simulink library "HEMERO"  (Simulink 3.00)
values from neighbouring files (symbols this model uses):
  K1 = 0.5    [ejh64.m]    (also in ejh65.m)
  K2 = 0.8    [ejh64.m]    (also in ejh65.m)
  x_camino = 0:0.01:10    [ejh64.m]    (also in ejh65.m)
  y_camino = x_camino.^2    [ejh64.m]    (also in ejh65.m)
undefined symbols (not defined in the file or in its folder): magnitude, nonlinear
libraries: simulink_extras x12, HEMERO x9, simulink3 x6, dspstat x4
(part 6 of 9)

== system HEMERO/Robots móviles/Control de robots móviles/Métodos basados en Teoría de Control/Seguimiento de trayectorias/Ejemplos/Ejemplo H.6.6/Seguimiento de trayectorias (Control lineal) ==
  note: w
  note: v
  v_r : Inport  Port=1  PortWidth=-1  SampleTime=-1  DataType=auto
      settings: SignalType=auto
  w_r : Inport  Port=2  PortWidth=-1  SampleTime=-1  DataType=auto
      settings: SignalType=auto
  Cambio de variable : Subsystem
  Configuración síncrona referencia : Subsystem
  Configuración síncrona robot real : Subsystem
  Control lineal : Subsystem
  Product : Product  Inputs=2  SaturateOnIntegerOverflow=on
  Sum : Sum  Inputs=-+  SaturateOnIntegerOverflow=on
  Sum1 : Sum  Inputs=+-  SaturateOnIntegerOverflow=on
  Trigonometric Function : Trigonometry  Operator=cos  OutputSignalType=auto
  v : Outport  Orientation=left  Port=1
  w : Outport  Orientation=left  Port=2
  x_ref : Outport  Port=3
  x : Outport  Port=4
  y_ref : Outport  Port=5
  y : Outport  Port=6
  phi_ref : Outport  Port=7
  phi : Outport  Port=8
  wires:
  Configuración síncrona robot real/3(phi) -> phi/1, Cambio de variable/6(phi)
  Configuración síncrona referencia/3(phi_r) -> phi_ref/1, Cambio de variable/5(phi_r)
  Configuración síncrona robot real/2(y) -> y/1, Cambio de variable/4(y)
  Configuración síncrona referencia/2(y_r) -> y_ref/1, Cambio de variable/3(y_r)
  Configuración síncrona robot real/1(x) -> x/1, Cambio de variable/2(x)
  Configuración síncrona referencia/1(x_r) -> x_ref/1, Cambio de variable/1(x_r)
  Cambio de variable/3(e3) -> Control lineal/3(e3), Trigonometric Function/1
  Cambio de variable/2(e2) -> Control lineal/2(e2)
  Cambio de variable/1(e1) -> Control lineal/1(e1)
  Control lineal/1(u1) -> Sum/1
  Control lineal/2(u2) -> Sum1/2
  Sum/1 -> v/1, Configuración síncrona robot real/1(v)
  Sum1/1 -> w/1, Configuración síncrona robot real/2(w)
  w_r/1 -> Sum1/1, Configuración síncrona referencia/2(w_r)
  Product/1 -> Sum/2
  Trigonometric Function/1 -> Product/1
  v_r/1 -> Control lineal/4(v_r), Product/2, Configuración síncrona referencia/1(v_r)

== system HEMERO/Robots móviles/Control de robots móviles/Métodos basados en Teoría de Control/Seguimiento de trayectorias/Ejemplos/Ejemplo H.6.7/Seguimiento de trayectorias (Control lineal con escalado de velocidad) ==
  note: v
  note: w
  v_r : Inport  Port=1  PortWidth=-1  SampleTime=-1  DataType=auto
      settings: SignalType=auto
  w_r : Inport  Port=2  PortWidth=-1  SampleTime=-1  DataType=auto
      settings: SignalType=auto
  Cambio de variable : Subsystem
  Configuración síncrona referencia : Subsystem
  Configuración síncrona robot real : Subsystem
  Control lineal con escalado de velocidad : Subsystem
  Product : Product  Inputs=2  SaturateOnIntegerOverflow=on
  Sum : Sum  Inputs=-+  SaturateOnIntegerOverflow=on
  Sum1 : Sum  Inputs=+-  SaturateOnIntegerOverflow=on
  Trigonometric Function : Trigonometry  Operator=cos  OutputSignalType=auto
  v : Outport  Orientation=left  Port=1
  w : Outport  Orientation=left  Port=2
  x_ref : Outport  Port=3
  x : Outport  Port=4
  y_ref : Outport  Port=5
  y : Outport  Port=6
  phi_ref : Outport  Port=7
  phi : Outport  Port=8
  wires:
  v_r/1 -> Configuración síncrona referencia/1(v_r), Product/2, Control lineal con escalado de velocidad/4(v_r)
  Trigonometric Function/1 -> Product/1
  Product/1 -> Sum/2
  w_r/1 -> Configuración síncrona referencia/2(w_r), Sum1/1, Control lineal con escalado de velocidad/5(w_r)
  Sum1/1 -> Configuración síncrona robot real/2(w), w/1
  Sum/1 -> Configuración síncrona robot real/1(v), v/1
  Control lineal con escalado de velocidad/2(u2) -> Sum1/2
  Control lineal con escalado de velocidad/1(u1) -> Sum/1
  Cambio de variable/1(e1) -> Control lineal con escalado de velocidad/1(e1)
  Cambio de variable/2(e2) -> Control lineal con escalado de velocidad/2(e2)
  Cambio de variable/3(e3) -> Trigonometric Function/1, Control lineal con escalado de velocidad/3(e3)
  Configuración síncrona robot real/3(phi) -> Cambio de variable/6(phi), phi/1
  Configuración síncrona referencia/3(phi_r) -> Cambio de variable/5(phi_r), phi_ref/1
  Configuración síncrona robot real/2(y) -> Cambio de variable/4(y), y/1
  Configuración síncrona referencia/2(y_r) -> Cambio de variable/3(y_r), y_ref/1
  Configuración síncrona robot real/1(x) -> Cambio de variable/2(x), x/1
  Configuración síncrona referencia/1(x_r) -> Cambio de variable/1(x_r), x_ref/1

== system HEMERO/Robots móviles/Control de robots móviles/Métodos basados en Teoría de Control/Seguimiento de trayectorias/Ejemplos/Ejemplo H.6.8/Seguimiento de trayectorias (Control no lineal) ==
  note: v
  note: w
  v_r : Inport  Port=1  PortWidth=-1  SampleTime=-1  DataType=auto
      settings: SignalType=auto
  w_r : Inport  Port=2  PortWidth=-1  SampleTime=-1  DataType=auto
      settings: SignalType=auto
  " " : Trigonometry  Operator=cos  OutputSignalType=auto
  Cambio de variable : Subsystem
  Configuración síncrona referencia : Subsystem
  Configuración síncrona robot real : Subsystem
  Control no lineal : Subsystem
  Cálculo de K1 y K3 : Subsystem
  Product : Product  Inputs=2  SaturateOnIntegerOverflow=on
  Sum : Sum  Inputs=-+  SaturateOnIntegerOverflow=on
  Sum1 : Sum  Inputs=+-  SaturateOnIntegerOverflow=on
  v : Outport  Orientation=left  Port=1
  w : Outport  Orientation=left  Port=2
  x_ref : Outport  Port=3
  x : Outport  Port=4
  y_ref : Outport  Port=5
  y : Outport  Port=6
  phi_ref : Outport  Port=7
  phi : Outport  Port=8
  wires:
  v_r/1 -> Configuración síncrona referencia/1(v_r), Product/2, Control no lineal/4(v_r), Cálculo de K1 y K3/2(v_r)
  " "/1 -> Product/1
  Product/1 -> Sum/2
  w_r/1 -> Configuración síncrona referencia/2(w_r), Sum1/1, Cálculo de K1 y K3/1(w_r)
  Sum1/1 -> Configuración síncrona robot real/2(w), w/1
  Sum/1 -> Configuración síncrona robot real/1(v), v/1
  Control no lineal/2(u2) -> Sum1/2
  Control no lineal/1(u1) -> Sum/1
  Cambio de variable/1(e1) -> Control no lineal/1(e1)
  Cambio de variable/2(e2) -> Control no lineal/2(e2)
  Cambio de variable/3(e3) -> " "/1, Control no lineal/3(e3)
  Cálculo de K1 y K3/1(K1) -> Control no lineal/5(K1), Control no lineal/6(K3)
  Configuración síncrona robot real/3(phi) -> Cambio de variable/6(phi), phi/1
  Configuración síncrona referencia/1(x_r) -> Cambio de variable/1(x_r), x_ref/1
  Configuración síncrona robot real/1(x) -> Cambio de variable/2(x), x/1
  Configuración síncrona referencia/2(y_r) -> Cambio de variable/3(y_r), y_ref/1
  Configuración síncrona robot real/2(y) -> Cambio de variable/4(y), y/1
  Configuración síncrona referencia/3(phi_r) -> Cambio de variable/5(phi_r), phi_ref/1

== system HEMERO/Robots móviles/Control de robots móviles/Métodos basados en Teoría de Control/Seguimiento de trayectorias/Seguimiento de trayectorias (Control lineal con escalado de velocidad)/Cambio de variable/Cálculo de e1 ==
  x_r : Inport  Port=1  PortWidth=-1  SampleTime=-1  DataType=auto
      settings: SignalType=auto
  x : Inport  Port=2  PortWidth=-1  SampleTime=-1  DataType=auto
      settings: SignalType=auto
  y_r : Inport  Port=3  PortWidth=-1  SampleTime=-1  DataType=auto
      settings: SignalType=auto
  y : Inport  Port=4  PortWidth=-1  SampleTime=-1  DataType=auto
      settings: SignalType=auto
  phi : Inport  Port=5  PortWidth=-1  SampleTime=-1  DataType=auto
      settings: SignalType=auto
  Product : Product  Inputs=2  SaturateOnIntegerOverflow=on
  Product1 : Product  Inputs=2  SaturateOnIntegerOverflow=on
  Sum : Sum  Inputs=-+  SaturateOnIntegerOverflow=on
  Sum1 : Sum  Inputs=+-  SaturateOnIntegerOverflow=on
  Sum2 : Sum  Inputs=++  SaturateOnIntegerOverflow=on
  Trigonometric Function : Trigonometry  Operator=sin  OutputSignalType=auto
  Trigonometric Function1 : Trigonometry  Operator=cos  OutputSignalType=auto
  e1 : Outport  Port=1
  wires:
  Sum2/1 -> e1/1
  Product1/1 -> Sum2/2
  Product/1 -> Sum2/1
  Trigonometric Function1/1 -> Product1/2
  Sum1/1 -> Product1/1
  Trigonometric Function/1 -> Product/2
  Sum/1 -> Product/1
  phi/1 -> Trigonometric Function1/1, Trigonometric Function/1
  y/1 -> Sum1/2
  y_r/1 -> Sum1/1
  x/1 -> Sum/2
  x_r/1 -> Sum/1

== system HEMERO/Robots móviles/Control de robots móviles/Métodos basados en Teoría de Control/Seguimiento de trayectorias/Seguimiento de trayectorias (Control lineal con escalado de velocidad)/Cambio de variable/Cálculo de e2 ==
  x_r : Inport  Port=1  PortWidth=-1  SampleTime=-1  DataType=auto
      settings: SignalType=auto
  x : Inport  Port=2  PortWidth=-1  SampleTime=-1  DataType=auto
      settings: SignalType=auto
  y_r : Inport  Port=3  PortWidth=-1  SampleTime=-1  DataType=auto
      settings: SignalType=auto
  y : Inport  Port=4  PortWidth=-1  SampleTime=-1  DataType=auto
      settings: SignalType=auto
  phi : Inport  Port=5  PortWidth=-1  SampleTime=-1  DataType=auto
      settings: SignalType=auto
  Product : Product  Inputs=2  SaturateOnIntegerOverflow=on
  Product1 : Product  Inputs=2  SaturateOnIntegerOverflow=on
  Sum : Sum  Inputs=-+  SaturateOnIntegerOverflow=on
  Sum1 : Sum  Inputs=-+  SaturateOnIntegerOverflow=on
  Sum2 : Sum  Inputs=++  SaturateOnIntegerOverflow=on
  Trigonometric Function2 : Trigonometry  Operator=sin  OutputSignalType=auto
  Trigonometric Function3 : Trigonometry  Operator=cos  OutputSignalType=auto
  e2 : Outport  Port=1
  wires:
  Sum2/1 -> e2/1
  Product1/1 -> Sum2/2
  Product/1 -> Sum2/1
  Trigonometric Function2/1 -> Product1/2
  Sum1/1 -> Product1/1
  Trigonometric Function3/1 -> Product/2
  Sum/1 -> Product/1
  phi/1 -> Trigonometric Function2/1, Trigonometric Function3/1
  y/1 -> Sum1/2
  y_r/1 -> Sum1/1
  x/1 -> Sum/2
  x_r/1 -> Sum/1

== system HEMERO/Robots móviles/Control de robots móviles/Métodos basados en Teoría de Control/Seguimiento de trayectorias/Seguimiento de trayectorias (Control lineal con escalado de velocidad)/Cambio de variable/Cálculo de e3 ==
  phi_r : Inport  Port=1  PortWidth=-1  SampleTime=-1  DataType=auto
      settings: SignalType=auto
  phi : Inport  Port=2  PortWidth=-1  SampleTime=-1  DataType=auto
      settings: SignalType=auto
  Subsystem2 : Subsystem
      mask Description: Pasa phi gorro al intervalo -180,180
  suma : Sum  Inputs=+-  SaturateOnIntegerOverflow=on
  e3 : Outport  Port=1
  wires:
  Subsystem2/1(phi_go_mod) -> e3/1
  suma/1 -> Subsystem2/1(phi_gorro)
  phi_r/1 -> suma/1
  phi/1 -> suma/2

== system HEMERO/Robots móviles/Control de robots móviles/Métodos basados en Teoría de Control/Seguimiento de trayectorias/Seguimiento de trayectorias (Control lineal con escalado de velocidad)/Control lineal con escalado de velocidad/Cálculo de u1 ==
  e1 : Inport  Port=1  PortWidth=-1  SampleTime=-1  DataType=auto
      settings: SignalType=auto
  v_r : Inport  Port=2  PortWidth=-1  SampleTime=-1  DataType=auto
      settings: SignalType=auto
  w_r : Inport  Port=3  PortWidth=-1  SampleTime=-1  DataType=auto
      settings: SignalType=auto
  Constant : Constant  Value=b
  Fcn : Fcn  Expr=u^2
  Fcn1 : Fcn  Expr=u^2
  Fcn2 : Fcn  Expr=sqrt(u)
  Gain : Gain  Gain=-1  SaturateOnIntegerOverflow=on
  Gain1 : Gain  Gain=2*d  SaturateOnIntegerOverflow=on
  Product : Product  Inputs=2  SaturateOnIntegerOverflow=on
  Product1 : Product  Inputs=2  SaturateOnIntegerOverflow=on
  Sum : Sum  Inputs=++  SaturateOnIntegerOverflow=on
  u1 : Outport  Port=1
  K1 : Outport  Port=2
  wires:
  Gain1/1 -> K1/1, Product1/2
  Fcn2/1 -> Gain1/1
  Product1/1 -> u1/1
  Gain/1 -> Product1/1
  Sum/1 -> Fcn2/1
  Fcn/1 -> Sum/2
  Product/1 -> Sum/1
  Constant/1 -> Product/2
  Fcn1/1 -> Product/1
  v_r/1 -> Fcn1/1
  w_r/1 -> Fcn/1
  e1/1 -> Gain/1

== system HEMERO/Robots móviles/Control de robots móviles/Métodos basados en Teoría de Control/Seguimiento de trayectorias/Seguimiento de trayectorias (Control lineal con escalado de velocidad)/Control lineal con escalado de velocidad/Cálculo de u2  ==
  note: K2
  e2 : Inport  Port=1  PortWidth=-1  SampleTime=-1  DataType=auto
      settings: SignalType=auto
  e3 : Inport  Port=2  PortWidth=-1  SampleTime=-1  DataType=auto
      settings: SignalType=auto
  v_r : Inport  Port=3  PortWidth=-1  SampleTime=-1  DataType=auto
      settings: SignalType=auto
  K3 : Inport  Port=4  PortWidth=-1  SampleTime=-1  DataType=auto
      settings: SignalType=auto
  Abs : Abs
  Gain1 : Gain  Gain=-1  SaturateOnIntegerOverflow=on
  Gain2 : Gain  Gain=b  SaturateOnIntegerOverflow=on
  Product : Product  Inputs=2  SaturateOnIntegerOverflow=on
  Product1 : Product  Inputs=2  SaturateOnIntegerOverflow=on
  Product3 : Product  Inputs=2  SaturateOnIntegerOverflow=on
  Sign : Signum
  Sum : Sum  Inputs=+-  SaturateOnIntegerOverflow=on
  u2 : Outport  Port=1
  wires:
  K3/1 -> Product3/2
  Product3/1 -> Sum/2
  Sum/1 -> u2/1
  e3/1 -> Product3/1
  Product1/1 -> Sum/1
  Gain2/1 -> Product1/2
  Gain1/1 -> Product1/1
  Abs/1 -> Gain2/1
  v_r/1 -> Abs/1, Sign/1
  Product/1 -> Gain1/1
  e2/1 -> Product/1
  Sign/1 -> Product/2

== system HEMERO/Robots móviles/Control de robots móviles/Métodos basados en Teoría de Control/Seguimiento de trayectorias/Seguimiento de trayectorias (Control lineal)/Cambio de variable/Cálculo de e1 ==
  x_r : Inport  Port=1  PortWidth=-1  SampleTime=-1  DataType=auto
      settings: SignalType=auto
  x : Inport  Port=2  PortWidth=-1  SampleTime=-1  DataType=auto
      settings: SignalType=auto
  y_r : Inport  Port=3  PortWidth=-1  SampleTime=-1  DataType=auto
      settings: SignalType=auto
  y : Inport  Port=4  PortWidth=-1  SampleTime=-1  DataType=auto
      settings: SignalType=auto
  phi : Inport  Port=5  PortWidth=-1  SampleTime=-1  DataType=auto
      settings: SignalType=auto
  Product : Product  Inputs=2  SaturateOnIntegerOverflow=on
  Product1 : Product  Inputs=2  SaturateOnIntegerOverflow=on
  Sum : Sum  Inputs=-+  SaturateOnIntegerOverflow=on
  Sum1 : Sum  Inputs=+-  SaturateOnIntegerOverflow=on
  Sum2 : Sum  Inputs=++  SaturateOnIntegerOverflow=on
  Trigonometric Function : Trigonometry  Operator=sin  OutputSignalType=auto
  Trigonometric Function1 : Trigonometry  Operator=cos  OutputSignalType=auto
  e1 : Outport  Port=1
  wires:
  Sum2/1 -> e1/1
  Product1/1 -> Sum2/2
  Product/1 -> Sum2/1
  Trigonometric Function1/1 -> Product1/2
  Sum1/1 -> Product1/1
  Trigonometric Function/1 -> Product/2
  Sum/1 -> Product/1
  phi/1 -> Trigonometric Function1/1, Trigonometric Function/1
  y/1 -> Sum1/2
  y_r/1 -> Sum1/1
  x/1 -> Sum/2
  x_r/1 -> Sum/1

== system HEMERO/Robots móviles/Control de robots móviles/Métodos basados en Teoría de Control/Seguimiento de trayectorias/Seguimiento de trayectorias (Control lineal)/Cambio de variable/Cálculo de e2 ==
  x_r : Inport  Port=1  PortWidth=-1  SampleTime=-1  DataType=auto
      settings: SignalType=auto
  x : Inport  Port=2  PortWidth=-1  SampleTime=-1  DataType=auto
      settings: SignalType=auto
  y_r : Inport  Port=3  PortWidth=-1  SampleTime=-1  DataType=auto
      settings: SignalType=auto
  y : Inport  Port=4  PortWidth=-1  SampleTime=-1  DataType=auto
      settings: SignalType=auto
  phi : Inport  Port=5  PortWidth=-1  SampleTime=-1  DataType=auto
      settings: SignalType=auto
  Product : Product  Inputs=2  SaturateOnIntegerOverflow=on
  Product1 : Product  Inputs=2  SaturateOnIntegerOverflow=on
  Sum : Sum  Inputs=-+  SaturateOnIntegerOverflow=on
  Sum1 : Sum  Inputs=-+  SaturateOnIntegerOverflow=on
  Sum2 : Sum  Inputs=++  SaturateOnIntegerOverflow=on
  Trigonometric Function2 : Trigonometry  Operator=sin  OutputSignalType=auto
  Trigonometric Function3 : Trigonometry  Operator=cos  OutputSignalType=auto
  e2 : Outport  Port=1
  wires:
  Sum2/1 -> e2/1
  Product1/1 -> Sum2/2
  Product/1 -> Sum2/1
  Trigonometric Function2/1 -> Product1/2
  Sum1/1 -> Product1/1
  Trigonometric Function3/1 -> Product/2
  Sum/1 -> Product/1
  phi/1 -> Trigonometric Function2/1, Trigonometric Function3/1
  y/1 -> Sum1/2
  y_r/1 -> Sum1/1
  x/1 -> Sum/2
  x_r/1 -> Sum/1

== system HEMERO/Robots móviles/Control de robots móviles/Métodos basados en Teoría de Control/Seguimiento de trayectorias/Seguimiento de trayectorias (Control lineal)/Cambio de variable/Cálculo de e3 ==
  phi_r : Inport  Port=1  PortWidth=-1  SampleTime=-1  DataType=auto
      settings: SignalType=auto
  phi : Inport  Port=2  PortWidth=-1  SampleTime=-1  DataType=auto
      settings: SignalType=auto
  Subsystem2 : Subsystem
      mask Description: Pasa phi gorro al intervalo -180,180
  suma : Sum  Inputs=+-  SaturateOnIntegerOverflow=on
  e3 : Outport  Port=1
  wires:
  Subsystem2/1(phi_go_mod) -> e3/1
  suma/1 -> Subsystem2/1(phi_gorro)
  phi_r/1 -> suma/1
  phi/1 -> suma/2

== system HEMERO/Robots móviles/Control de robots móviles/Métodos basados en Teoría de Control/Seguimiento de trayectorias/Seguimiento de trayectorias (Control lineal)/Control lineal/Cálculo de u1 ==
  e1 : Inport  Port=1  PortWidth=-1  SampleTime=-1  DataType=auto
      settings: SignalType=auto
  Gain : Gain  Gain=-K1  SaturateOnIntegerOverflow=on
  u1 : Outport  Port=1
  wires:
  Gain/1 -> u1/1
  e1/1 -> Gain/1

== system HEMERO/Robots móviles/Control de robots móviles/Métodos basados en Teoría de Control/Seguimiento de trayectorias/Seguimiento de trayectorias (Control lineal)/Control lineal/Cálculo de u2  ==
  e2 : Inport  Port=1  PortWidth=-1  SampleTime=-1  DataType=auto
      settings: SignalType=auto
  e3 : Inport  Port=2  PortWidth=-1  SampleTime=-1  DataType=auto
      settings: SignalType=auto
  v_r : Inport  Port=3  PortWidth=-1  SampleTime=-1  DataType=auto
      settings: SignalType=auto
  Gain1 : Gain  Gain=-K2  SaturateOnIntegerOverflow=on
  Gain3 : Gain  Gain=-K3  SaturateOnIntegerOverflow=on
  Product1 : Product  Inputs=2  SaturateOnIntegerOverflow=on
  Sign : Signum
  Sum : Sum  Inputs=++  SaturateOnIntegerOverflow=on
  u2 : Outport  Port=1
  wires:
  Sign/1 -> Product1/2
  v_r/1 -> Sign/1
  e2/1 -> Gain1/1
  Gain3/1 -> Sum/2
  e3/1 -> Gain3/1
  Sum/1 -> u2/1
  Product1/1 -> Sum/1
  Gain1/1 -> Product1/1

== system HEMERO/Robots móviles/Control de robots móviles/Métodos basados en Teoría de Control/Seguimiento de trayectorias/Seguimiento de trayectorias (Control no lineal)/Cambio de variable/Cálculo de e1 ==
  x_r : Inport  Port=1  PortWidth=-1  SampleTime=-1  DataType=auto
      settings: SignalType=auto
  x : Inport  Port=2  PortWidth=-1  SampleTime=-1  DataType=auto
      settings: SignalType=auto
  y_r : Inport  Port=3  PortWidth=-1  SampleTime=-1  DataType=auto
      settings: SignalType=auto
  y : Inport  Port=4  PortWidth=-1  SampleTime=-1  DataType=auto
      settings: SignalType=auto
  phi : Inport  Port=5  PortWidth=-1  SampleTime=-1  DataType=auto
      settings: SignalType=auto
  Product : Product  Inputs=2  SaturateOnIntegerOverflow=on
  Product1 : Product  Inputs=2  SaturateOnIntegerOverflow=on
  Sum : Sum  Inputs=-+  SaturateOnIntegerOverflow=on
  Sum1 : Sum  Inputs=+-  SaturateOnIntegerOverflow=on
  Sum2 : Sum  Inputs=++  SaturateOnIntegerOverflow=on
  Trigonometric Function : Trigonometry  Operator=sin  OutputSignalType=auto
  Trigonometric Function1 : Trigonometry  Operator=cos  OutputSignalType=auto
  e1 : Outport  Port=1
  wires:
  Sum2/1 -> e1/1
  Product1/1 -> Sum2/2
  Product/1 -> Sum2/1
  Trigonometric Function1/1 -> Product1/2
  Sum1/1 -> Product1/1
  Trigonometric Function/1 -> Product/2
  Sum/1 -> Product/1
  phi/1 -> Trigonometric Function1/1, Trigonometric Function/1
  y/1 -> Sum1/2
  y_r/1 -> Sum1/1
  x/1 -> Sum/2
  x_r/1 -> Sum/1

== system HEMERO/Robots móviles/Control de robots móviles/Métodos basados en Teoría de Control/Seguimiento de trayectorias/Seguimiento de trayectorias (Control no lineal)/Cambio de variable/Cálculo de e2 ==
  x_r : Inport  Port=1  PortWidth=-1  SampleTime=-1  DataType=auto
      settings: SignalType=auto
  x : Inport  Port=2  PortWidth=-1  SampleTime=-1  DataType=auto
      settings: SignalType=auto
  y_r : Inport  Port=3  PortWidth=-1  SampleTime=-1  DataType=auto
      settings: SignalType=auto
  y : Inport  Port=4  PortWidth=-1  SampleTime=-1  DataType=auto
      settings: SignalType=auto
  phi : Inport  Port=5  PortWidth=-1  SampleTime=-1  DataType=auto
      settings: SignalType=auto
  Product : Product  Inputs=2  SaturateOnIntegerOverflow=on
  Product1 : Product  Inputs=2  SaturateOnIntegerOverflow=on
  Sum : Sum  Inputs=-+  SaturateOnIntegerOverflow=on
  Sum1 : Sum  Inputs=-+  SaturateOnIntegerOverflow=on
  Sum2 : Sum  Inputs=++  SaturateOnIntegerOverflow=on
  Trigonometric Function2 : Trigonometry  Operator=sin  OutputSignalType=auto
  Trigonometric Function3 : Trigonometry  Operator=cos  OutputSignalType=auto
  e2 : Outport  Port=1
  wires:
  Sum2/1 -> e2/1
  Product1/1 -> Sum2/2
  Product/1 -> Sum2/1
  Trigonometric Function2/1 -> Product1/2
  Sum1/1 -> Product1/1
  Trigonometric Function3/1 -> Product/2
  Sum/1 -> Product/1
  phi/1 -> Trigonometric Function2/1, Trigonometric Function3/1
  y/1 -> Sum1/2
  y_r/1 -> Sum1/1
  x/1 -> Sum/2
  x_r/1 -> Sum/1

== system HEMERO/Robots móviles/Control de robots móviles/Métodos basados en Teoría de Control/Seguimiento de trayectorias/Seguimiento de trayectorias (Control no lineal)/Cambio de variable/Cálculo de e3 ==
  phi_r : Inport  Port=1  PortWidth=-1  SampleTime=-1  DataType=auto
      settings: SignalType=auto
  phi : Inport  Port=2  PortWidth=-1  SampleTime=-1  DataType=auto
      settings: SignalType=auto
  Subsystem2 : Subsystem
      mask Description: Pasa phi gorro al intervalo -180,180
  suma : Sum  Inputs=+-  SaturateOnIntegerOverflow=on
  e3 : Outport  Port=1
  wires:
  Subsystem2/1(phi_go_mod) -> e3/1
  suma/1 -> Subsystem2/1(phi_gorro)
  phi_r/1 -> suma/1
  phi/1 -> suma/2

== system HEMERO/Robots móviles/Control de robots móviles/Métodos basados en Teoría de Control/Seguimiento de trayectorias/Seguimiento de trayectorias (Control no lineal)/Control no lineal/Cálculo de u1 ==
  e1 : Inport  Port=1  PortWidth=-1  SampleTime=-1  DataType=auto
      settings: SignalType=auto
  K1 : Inport  Port=2  PortWidth=-1  SampleTime=-1  DataType=auto
      settings: SignalType=auto
  Gain : Gain  Gain=-1  SaturateOnIntegerOverflow=on
  Product : Product  Inputs=2  SaturateOnIntegerOverflow=on
  u1 : Outport  Port=1
  wires:
  Gain/1 -> Product/2
  K1/1 -> Gain/1
  Product/1 -> u1/1
  e1/1 -> Product/1

== system HEMERO/Robots móviles/Control de robots móviles/Métodos basados en Teoría de Control/Seguimiento de trayectorias/Seguimiento de trayectorias (Control no lineal)/Control no lineal/Cálculo de u2  ==
  e2 : Inport  Port=1  PortWidth=-1  SampleTime=-1  DataType=auto
      settings: SignalType=auto
  e3 : Inport  Port=2  PortWidth=-1  SampleTime=-1  DataType=auto
      settings: SignalType=auto
  v_r : Inport  Port=3  PortWidth=-1  SampleTime=-1  DataType=auto
      settings: SignalType=auto
  K3 : Inport  Port=4  PortWidth=-1  SampleTime=-1  DataType=auto
      settings: SignalType=auto
  Gain1 : Gain  Gain=-K2  SaturateOnIntegerOverflow=on
  Gain2 : Gain  Gain=-1  SaturateOnIntegerOverflow=on
  MATLAB Fcn : MATLABFcn  MATLABFcn=nonlinear(u)  OutputWidth=-1  OutputSignalType=auto
  Product1 : Product  Inputs=3  SaturateOnIntegerOverflow=on
  Product2 : Product  Inputs=2  SaturateOnIntegerOverflow=on
  Sum : Sum  Inputs=++  SaturateOnIntegerOverflow=on
  u2 : Outport  Port=1
  wires:
  e3/1 -> Product2/1, MATLAB Fcn/1
  v_r/1 -> Product1/2
  Product2/1 -> Sum/2
  Gain2/1 -> Product2/2
  K3/1 -> Gain2/1
  e2/1 -> Gain1/1
  Sum/1 -> u2/1
  Product1/1 -> Sum/1
  Gain1/1 -> Product1/1
  MATLAB Fcn/1 -> Product1/3

== system HEMERO/Robots móviles/Control de robots móviles/Métodos basados en Teoría de Control/Seguimiento de caminos/Ejemplos/Ejemplo H.6.4/Seguimiento de caminos (control lineal)/Configuracion síncrona ==
  v : Inport  Port=1  PortWidth=-1  SampleTime=-1  DataType=auto
      settings: SignalType=auto
  w : Inport  Port=2  PortWidth=-1  SampleTime=-1  DataType=auto
      settings: SignalType=auto
  Fcn : Fcn  Expr=-sin(u)
  Fcn1 : Fcn  Expr=cos(u)
  Integrator : Integrator  ExternalReset=none  InitialConditionSource=internal  InitialCondition=phi_inicial  LimitOutput=off  UpperSaturationLimit=inf  LowerSaturationLimit=-inf  ShowSaturationPort=off  ShowStatePort=off  AbsoluteTolerance=auto
  Integrator1 : Integrator  ExternalReset=none  InitialConditionSource=internal  InitialCondition=x_inicial  LimitOutput=off  UpperSaturationLimit=inf  LowerSaturationLimit=-inf  ShowSaturationPort=off  ShowStatePort=off  AbsoluteTolerance=auto
  Integrator2 : Integrator  ExternalReset=none  InitialConditionSource=internal  InitialCondition=y_inicial  LimitOutput=off  UpperSaturationLimit=inf  LowerSaturationLimit=-inf  ShowSaturationPort=off  ShowStatePort=off  AbsoluteTolerance=auto
  Product : Product  Inputs=2  SaturateOnIntegerOverflow=on
  Product1 : Product  Inputs=2  SaturateOnIntegerOverflow=on
  x_vehículo : Outport  Port=1
  y_vehículo : Outport  Port=2
  phi_vehículo : Outport  Port=3
  wires:
  Fcn1/1 -> Product1/2
  w/1 -> Integrator/1
  v/1 -> Product1/1, Product/1
  Integrator2/1 -> y_vehículo/1
  Integrator1/1 -> x_vehículo/1
  Integrator/1 -> phi_vehículo/1, Fcn1/1, Fcn/1
  Fcn/1 -> Product/2
  Product/1 -> Integrator1/1
  Product1/1 -> Integrator2/1

== system HEMERO/Robots móviles/Control de robots móviles/Métodos basados en Teoría de Control/Seguimiento de caminos/Ejemplos/Ejemplo H.6.4/Seguimiento de caminos (control lineal)/Controlador lineal ==
  fi_gorro : Inport  Port=1  PortWidth=-1  SampleTime=-1  DataType=auto
      settings: SignalType=auto
  v : Inport  Port=2  PortWidth=-1  SampleTime=-1  DataType=auto
      settings: SignalType=auto
  epsilon : Inport  Port=3  PortWidth=-1  SampleTime=-1  DataType=auto
      settings: SignalType=auto
  Abs : Abs
  Gain : Gain  Gain=K1  SaturateOnIntegerOverflow=on
  Gain1 : Gain  Gain=K2  SaturateOnIntegerOverflow=on
  Product : Product  Inputs=2  SaturateOnIntegerOverflow=on
  Product1 : Product  Inputs=2  SaturateOnIntegerOverflow=on
  Sum : Sum  Inputs=--  SaturateOnIntegerOverflow=on
  u_cont : Outport  Port=1  InitialOutput=0
  wires:
  Gain/1 -> Product/1
  v/1 -> Product/2, Abs/1
  Gain1/1 -> Product1/1
  Abs/1 -> Product1/2
  Product/1 -> Sum/1
  Product1/1 -> Sum/2
  epsilon/1 -> Gain/1
  Sum/1 -> u_cont/1
  fi_gorro/1 -> Gain1/1

== system HEMERO/Robots móviles/Control de robots móviles/Métodos basados en Teoría de Control/Seguimiento de caminos/Ejemplos/Ejemplo H.6.4/Seguimiento de caminos (control lineal)/Convertidor ==
  R_c : Inport  Port=1  PortWidth=-1  SampleTime=-1  DataType=auto
      settings: SignalType=auto
  fi_gorro : Inport  Port=2  PortWidth=-1  SampleTime=-1  DataType=auto
      settings: SignalType=auto
  v : Inport  Port=3  PortWidth=-1  SampleTime=-1  DataType=auto
      settings: SignalType=auto
  u_cont : Inport  Port=4  PortWidth=-1  SampleTime=-1  DataType=auto
      settings: SignalType=auto
  Constant : Constant  Value=1
  Gain : Gain  Gain=-1  SaturateOnIntegerOverflow=on
  Math Function : Math  Operator=reciprocal  OutputSignalType=auto
  Math Function1 : Math  Operator=reciprocal  OutputSignalType=auto
  Product : Product  Inputs=3  SaturateOnIntegerOverflow=on
  Product1 : Product  Inputs=3  SaturateOnIntegerOverflow=on
  Product2 : Product  Inputs=2  SaturateOnIntegerOverflow=on
  Sum : Sum  Inputs=++  SaturateOnIntegerOverflow=on
  Sum1 : Sum  Inputs=++  SaturateOnIntegerOverflow=on
  Trigonometric Function : Trigonometry  Operator=cos  OutputSignalType=auto
  Trigonometric Function1 : Trigonometry  Operator=sin  OutputSignalType=auto
  w : Outport  Port=1  InitialOutput=0
  wires:
  Math Function1/1 -> Gain/1, Product2/2
  R_c/1 -> Math Function1/1
  fi_gorro/1 -> Trigonometric Function/1, Trigonometric Function1/1
  Trigonometric Function1/1 -> Product1/1
  Gain/1 -> Product1/3
  Product1/1 -> Sum1/1
  Constant/1 -> Sum1/2
  Sum1/1 -> Math Function/1
  Trigonometric Function/1 -> Product/1
  v/1 -> Product1/2, Product/2
  Math Function/1 -> Product2/1
  Product/1 -> Sum/2
  u_cont/1 -> Sum/1
  Sum/1 -> w/1
  Product2/1 -> Product/3

== system HEMERO/Robots móviles/Control de robots móviles/Métodos basados en Teoría de Control/Seguimiento de caminos/Ejemplos/Ejemplo H.6.4/Seguimiento de caminos (control lineal)/Cálculo de parámetros ==
  x_camino : Inport  Port=1  PortWidth=-1  SampleTime=-1  DataType=auto
      settings: SignalType=auto
  y_camino : Inport  Port=2  PortWidth=-1  SampleTime=-1  DataType=auto
      settings: SignalType=auto
  x_vehiculo : Inport  Port=3  PortWidth=-1  SampleTime=-1  DataType=auto
      settings: SignalType=auto
  y_vehiculo : Inport  Port=4  PortWidth=-1  SampleTime=-1  DataType=auto
      settings: SignalType=auto
  phi_vehiculo : Inport  Port=5  PortWidth=-1  SampleTime=-1  DataType=auto
      settings: SignalType=auto
  Cálculo de phi gorro : Subsystem
  Degrees to Radians : simulink_extras/Transformations/Degrees to Radians
  Subsystem : Subsystem
  epsilon : Outport  Port=1
  fi_gorro : Outport  Port=2
  R_c : Outport  Port=3
  wires:
  x_camino/1 -> Subsystem/1(x_camino)
  y_camino/1 -> Subsystem/2(y_camino)
  y_vehiculo/1 -> Subsystem/4(y_vehiculo)
  x_vehiculo/1 -> Subsystem/3(x_vehiculo)
  Subsystem/3(R_c) -> R_c/1
  phi_vehiculo/1 -> Cálculo de phi gorro/1(fi_vehiculo)
  Degrees to Radians/1 -> fi_gorro/1
  Cálculo de phi gorro/1(fi_go_mo) -> Degrees to Radians/1
  Subsystem/1(distancia) -> epsilon/1
  Subsystem/2(indice) -> Cálculo de phi gorro/2(indice)

== system HEMERO/Robots móviles/Control de robots móviles/Métodos basados en Teoría de Control/Seguimiento de caminos/Ejemplos/Ejemplo H.6.5/Seguimiento de caminos (control no lineal)/  ==
  v : Inport  Port=1  PortWidth=-1  SampleTime=-1  DataType=auto
      settings: SignalType=auto
  Abs : Abs
  Gain : Gain  Gain=K2  SaturateOnIntegerOverflow=on
  k (v) : Outport  Port=1
  wires:
  Gain/1 -> k (v)/1
  Abs/1 -> Gain/1
  v/1 -> Abs/1

== system HEMERO/Robots móviles/Control de robots móviles/Métodos basados en Teoría de Control/Seguimiento de caminos/Ejemplos/Ejemplo H.6.5/Seguimiento de caminos (control no lineal)/Configuracion síncrona ==
  v : Inport  Port=1  PortWidth=-1  SampleTime=-1  DataType=auto
      settings: SignalType=auto
  w : Inport  Port=2  PortWidth=-1  SampleTime=-1  DataType=auto
      settings: SignalType=auto
  Fcn : Fcn  Expr=-sin(u)
  Fcn1 : Fcn  Expr=cos(u)
  Integrator : Integrator  ExternalReset=none  InitialConditionSource=internal  InitialCondition=phi_inicial  LimitOutput=off  UpperSaturationLimit=inf  LowerSaturationLimit=-inf  ShowSaturationPort=off  ShowStatePort=off  AbsoluteTolerance=auto
  Integrator1 : Integrator  ExternalReset=none  InitialConditionSource=internal  InitialCondition=x_inicial  LimitOutput=off  UpperSaturationLimit=inf  LowerSaturationLimit=-inf  ShowSaturationPort=off  ShowStatePort=off  AbsoluteTolerance=auto
  Integrator2 : Integrator  ExternalReset=none  InitialConditionSource=internal  InitialCondition=y_inicial  LimitOutput=off  UpperSaturationLimit=inf  LowerSaturationLimit=-inf  ShowSaturationPort=off  ShowStatePort=off  AbsoluteTolerance=auto
  Product : Product  Inputs=2  SaturateOnIntegerOverflow=on
  Product1 : Product  Inputs=2  SaturateOnIntegerOverflow=on
  x_vehículo : Outport  Port=1
  y_vehículo : Outport  Port=2
  phi_vehículo : Outport  Port=3
  wires:
  Fcn1/1 -> Product1/2
  w/1 -> Integrator/1
  v/1 -> Product1/1, Product/1
  Integrator2/1 -> y_vehículo/1
  Integrator1/1 -> x_vehículo/1
  Integrator/1 -> phi_vehículo/1, Fcn1/1, Fcn/1
  Fcn/1 -> Product/2
  Product/1 -> Integrator1/1
  Product1/1 -> Integrator2/1

== system HEMERO/Robots móviles/Control de robots móviles/Métodos basados en Teoría de Control/Seguimiento de caminos/Ejemplos/Ejemplo H.6.5/Seguimiento de caminos (control no lineal)/Controlador no lineal ==
  phi_gorro : Inport  Port=1  PortWidth=-1  SampleTime=-1  DataType=auto
      settings: SignalType=auto
  v : Inport  Port=2  PortWidth=-1  SampleTime=-1  DataType=auto
      settings: SignalType=auto
  epsilon : Inport  Port=3  PortWidth=-1  SampleTime=-1  DataType=auto
      settings: SignalType=auto
  k (v) : Inport  Port=4  PortWidth=-1  SampleTime=-1  DataType=auto
      settings: SignalType=auto
  Gain : Gain  Gain=K1  SaturateOnIntegerOverflow=on
  MATLAB Fcn : MATLABFcn  MATLABFcn=nonlinear(u)  OutputWidth=-1  OutputSignalType=auto
  Product : Product  Inputs=3  SaturateOnIntegerOverflow=on
  Product1 : Product  Inputs=2  SaturateOnIntegerOverflow=on
  Sum : Sum  Inputs=--  SaturateOnIntegerOverflow=on
  u_cont : Outport  Port=1  InitialOutput=0
  wires:
  k (v)/1 -> Product1/2
  v/1 -> Product/2
  phi_gorro/1 -> Product1/1, MATLAB Fcn/1
  Gain/1 -> Product/1
  Product/1 -> Sum/1
  Product1/1 -> Sum/2
  epsilon/1 -> Gain/1
  Sum/1 -> u_cont/1
  MATLAB Fcn/1 -> Product/3

== system HEMERO/Robots móviles/Control de robots móviles/Métodos basados en Teoría de Control/Seguimiento de caminos/Ejemplos/Ejemplo H.6.5/Seguimiento de caminos (control no lineal)/Convertidor ==
  R_c : Inport  Port=1  PortWidth=-1  SampleTime=-1  DataType=auto
      settings: SignalType=auto
  fi_gorro : Inport  Port=2  PortWidth=-1  SampleTime=-1  DataType=auto
      settings: SignalType=auto
  v : Inport  Port=3  PortWidth=-1  SampleTime=-1  DataType=auto
      settings: SignalType=auto
  u_cont : Inport  Port=4  PortWidth=-1  SampleTime=-1  DataType=auto
      settings: SignalType=auto
  Constant : Constant  Value=1
  Gain : Gain  Gain=-1  SaturateOnIntegerOverflow=on
  Math Function : Math  Operator=reciprocal  OutputSignalType=auto
  Math Function1 : Math  Operator=reciprocal  OutputSignalType=auto
  Product : Product  Inputs=3  SaturateOnIntegerOverflow=on
  Product1 : Product  Inputs=3  SaturateOnIntegerOverflow=on
  Product2 : Product  Inputs=2  SaturateOnIntegerOverflow=on
  Sum : Sum  Inputs=++  SaturateOnIntegerOverflow=on
  Sum1 : Sum  Inputs=++  SaturateOnIntegerOverflow=on
  Trigonometric Function : Trigonometry  Operator=cos  OutputSignalType=auto
  Trigonometric Function1 : Trigonometry  Operator=sin  OutputSignalType=auto
  w : Outport  Port=1  InitialOutput=0
  wires:
  Math Function1/1 -> Gain/1, Product2/2
  R_c/1 -> Math Function1/1
  fi_gorro/1 -> Trigonometric Function/1, Trigonometric Function1/1
  Trigonometric Function1/1 -> Product1/1
  Gain/1 -> Product1/3
  Product1/1 -> Sum1/1
  Constant/1 -> Sum1/2
  Sum1/1 -> Math Function/1
  Trigonometric Function/1 -> Product/1
  v/1 -> Product1/2, Product/2
  Math Function/1 -> Product2/1
  Product/1 -> Sum/2
  u_cont/1 -> Sum/1
  Sum/1 -> w/1
  Product2/1 -> Product/3

== system HEMERO/Robots móviles/Control de robots móviles/Métodos basados en Teoría de Control/Seguimiento de caminos/Ejemplos/Ejemplo H.6.5/Seguimiento de caminos (control no lineal)/Cálculo de parámetros ==
  x_camino : Inport  Port=1  PortWidth=-1  SampleTime=-1  DataType=auto
      settings: SignalType=auto
  y_camino : Inport  Port=2  PortWidth=-1  SampleTime=-1  DataType=auto
      settings: SignalType=auto
  x_vehiculo : Inport  Port=3  PortWidth=-1  SampleTime=-1  DataType=auto
      settings: SignalType=auto
  y_vehiculo : Inport  Port=4  PortWidth=-1  SampleTime=-1  DataType=auto
      settings: SignalType=auto
  phi_vehiculo : Inport  Port=5  PortWidth=-1  SampleTime=-1  DataType=auto
      settings: SignalType=auto
  Cálculo de phi gorro : Subsystem
  Degrees to Radians : simulink_extras/Transformations/Degrees to Radians
  Subsystem : Subsystem
  epsilon : Outport  Port=1
  fi_gorro : Outport  Port=2
  R_c : Outport  Port=3
  wires:
  x_camino/1 -> Subsystem/1(x_camino)
  y_camino/1 -> Subsystem/2(y_camino)
  y_vehiculo/1 -> Subsystem/4(y_vehiculo)
  x_vehiculo/1 -> Subsystem/3(x_vehiculo)
  Subsystem/3(R_c) -> R_c/1
  phi_vehiculo/1 -> Cálculo de phi gorro/1(fi_vehiculo)
  Degrees to Radians/1 -> fi_gorro/1
  Cálculo de phi gorro/1(fi_go_mo) -> Degrees to Radians/1
  Subsystem/1(distancia) -> epsilon/1
  Subsystem/2(indice) -> Cálculo de phi gorro/2(indice)

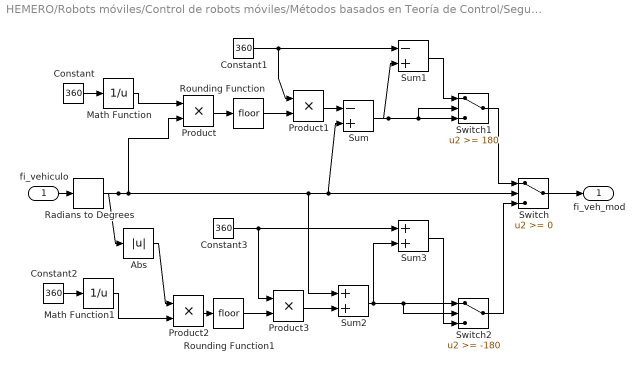
== system HEMERO/Robots móviles/Control de robots móviles/Métodos basados en Teoría de Control/Seguimiento de caminos/Seguimiento de caminos (control lineal)/Cálculo de parámetros/Cálculo de phi gorro/Subsystem ==
  fi_vehiculo : Inport  Port=1  PortWidth=-1  SampleTime=-1  DataType=auto
      settings: SignalType=auto
  Abs : Abs
  Constant{,1..3} (4 alike) : Constant  Value=360
  Math Function : Math  Operator=reciprocal  OutputSignalType=auto
  Math Function1 : Math  Operator=reciprocal  OutputSignalType=auto
  Product{,1..3} (4 alike) : Product  Inputs=2  SaturateOnIntegerOverflow=on
  Radians to Degrees : simulink_extras/Transformations/Radians to Degrees
  Rounding Function : Rounding  Operator=floor
  Rounding Function1 : Rounding  Operator=floor
  Sum : Sum  Inputs=-+  SaturateOnIntegerOverflow=on
  Sum1 : Sum  Inputs=-+  SaturateOnIntegerOverflow=on
  Sum2 : Sum  Inputs=++  SaturateOnIntegerOverflow=on
  Sum3 : Sum  Inputs=++  SaturateOnIntegerOverflow=on
  Switch : Switch  Threshold=0
  Switch1 : Switch  Threshold=180
  Switch2 : Switch  Threshold=-180
  fi_veh_mod : Outport  Port=1
  wires:
  Switch/1 -> fi_veh_mod/1
  Switch1/1 -> Switch/1
  Math Function/1 -> Product/1
  Constant/1 -> Math Function/1
  Product/1 -> Rounding Function/1
  Rounding Function/1 -> Product1/2
  Product1/1 -> Sum/1
  Constant1/1 -> Product1/1, Sum1/1
  Sum/1 -> Sum1/2, Switch1/3, Switch1/2
  Sum1/1 -> Switch1/1
  Constant3/1 -> Product3/1, Sum3/1
  Switch2/1 -> Switch/3
  Rounding Function1/1 -> Product3/2
  Product3/1 -> Sum2/2
  Constant2/1 -> Math Function1/1
  Math Function1/1 -> Product2/2
  Product2/1 -> Rounding Function1/1
  Sum3/1 -> Switch2/3
  Sum2/1 -> Sum3/2, Switch2/1, Switch2/2
  Abs/1 -> Product2/1
  fi_vehiculo/1 -> Radians to Degrees/1
  Radians to Degrees/1 -> Product/2, Switch/2, Sum/2, Sum2/1, Abs/1

== system HEMERO/Robots móviles/Control de robots móviles/Métodos basados en Teoría de Control/Seguimiento de caminos/Seguimiento de caminos (control lineal)/Cálculo de parámetros/Cálculo de phi gorro/Subsystem1 ==
  indice : Inport  Port=1  PortWidth=-1  SampleTime=-1  DataType=auto
      settings: SignalType=auto
  Constant : Constant  Value=90
  Constant1 : Constant  Value=360
  Look-Up Table : Lookup  InputValues=1:length(der_x)  OutputValues=der_x(1:length(der_x))
  Look-Up Table1 : Lookup  InputValues=1:length(der_y)  OutputValues=der_y(1:length(der_y))
  Radians to Degrees : simulink_extras/Transformations/Radians to Degrees
  Sum : Sum  Inputs=+-  SaturateOnIntegerOverflow=on
  Sum1 : Sum  Inputs=++  SaturateOnIntegerOverflow=on
  Switch : Switch  Threshold=-180
  Trigonometric Function : Trigonometry  Operator=atan2  OutputSignalType=auto
  fi_camino : Outport  Port=1
  wires:
  Look-Up Table1/1 -> Trigonometric Function/1
  Look-Up Table/1 -> Trigonometric Function/2
  Trigonometric Function/1 -> Radians to Degrees/1
  Radians to Degrees/1 -> Sum/1
  Constant/1 -> Sum/2
  Constant1/1 -> Sum1/2
  Sum/1 -> Switch/1, Sum1/1, Switch/2
  Sum1/1 -> Switch/3
  Switch/1 -> fi_camino/1
  indice/1 -> Look-Up Table1/1, Look-Up Table/1

== system HEMERO/Robots móviles/Control de robots móviles/Métodos basados en Teoría de Control/Seguimiento de caminos/Seguimiento de caminos (control lineal)/Cálculo de parámetros/Cálculo de phi gorro/Subsystem2 ==
  fi_gorro : Inport  Port=1  PortWidth=-1  SampleTime=-1  DataType=auto
      settings: SignalType=auto
  Constant1 : Constant  Value=360
  Constant2 : Constant  Value=360
  Sum1 : Sum  Inputs=-+  SaturateOnIntegerOverflow=on
  Sum2 : Sum  Inputs=++  SaturateOnIntegerOverflow=on
  Switch : Switch  Threshold=180
  Switch1 : Switch  Threshold=0
  Switch2 : Switch  Threshold=-180
  fi_go_mo : Outport  Port=1
  wires:
  Switch1/1 -> fi_go_mo/1
  Switch/1 -> Switch1/1
  Switch2/1 -> Switch1/3
  Constant1/1 -> Sum1/1
  Sum1/1 -> Switch/1
  Sum2/1 -> Switch2/3
  fi_gorro/1 -> Sum1/2, Switch1/2, Switch/3, Switch/2, Switch2/1, Switch2/2, Sum2/1
  Constant2/1 -> Sum2/2

== system HEMERO/Robots móviles/Control de robots móviles/Métodos basados en Teoría de Control/Seguimiento de caminos/Seguimiento de caminos (control lineal)/Cálculo de parámetros/Subsystem/Parametros de Curvatura ==
  x_1 : Inport  Port=1  PortWidth=-1  SampleTime=-1  DataType=auto
      settings: SignalType=auto
  x_2 : Inport  Port=2  PortWidth=-1  SampleTime=-1  DataType=auto
      settings: SignalType=auto
  x_3 : Inport  Port=3  PortWidth=-1  SampleTime=-1  DataType=auto
      settings: SignalType=auto
  y_1 : Inport  Port=4  PortWidth=-1  SampleTime=-1  DataType=auto
      settings: SignalType=auto
  y_2 : Inport  Port=5  PortWidth=-1  SampleTime=-1  DataType=auto
      settings: SignalType=auto
  y_3 : Inport  Port=6  PortWidth=-1  SampleTime=-1  DataType=auto
      settings: SignalType=auto
  Radio de  Curvatura : Subsystem
  coordenada x c. curvatura : Subsystem
  coordenada y c. curvatura : Subsystem
  x_g : Outport  Port=1  InitialOutput=0
  y_g : Outport  Port=2  InitialOutput=0
  R_c : Outport  Port=3  InitialOutput=0
  wires:
  Radio de  Curvatura/1(R_c) -> R_c/1
  coordenada y c. curvatura/1(y_g) -> y_g/1, Radio de  Curvatura/3(y_g)
  coordenada x c. curvatura/1(x_g) -> x_g/1, Radio de  Curvatura/1(x_g)
  x_1/1 -> coordenada x c. curvatura/1(x_1), coordenada y c. curvatura/1(x_1), Radio de  Curvatura/2(x_1)
  x_2/1 -> coordenada x c. curvatura/2(x_2), coordenada y c. curvatura/2(x_2)
  x_3/1 -> coordenada x c. curvatura/3(x_3), coordenada y c. curvatura/3(x_3)
  y_1/1 -> coordenada y c. curvatura/4(y_1), coordenada x c. curvatura/4(y_1), Radio de  Curvatura/4(y_1)
  y_2/1 -> coordenada x c. curvatura/5(y_2), coordenada y c. curvatura/5(y_2)
  y_3/1 -> coordenada y c. curvatura/6(y_3), coordenada x c. curvatura/6(y_3)

== system HEMERO/Robots móviles/Control de robots móviles/Métodos basados en Teoría de Control/Seguimiento de caminos/Seguimiento de caminos (control lineal)/Cálculo de parámetros/Subsystem/Subsystem ==
  x : Inport  Port=1  PortWidth=-1  SampleTime=-1  DataType=auto
      settings: SignalType=auto
  y : Inport  Port=2  PortWidth=-1  SampleTime=-1  DataType=auto
      settings: SignalType=auto
  x_g : Inport  Port=3  PortWidth=-1  SampleTime=-1  DataType=auto
      settings: SignalType=auto
  y_g : Inport  Port=4  PortWidth=-1  SampleTime=-1  DataType=auto
      settings: SignalType=auto
  Math Function2 : Math  Operator=sqrt  OutputSignalType=auto
  Math Function3 : Math  Operator=square  OutputSignalType=auto
  Math Function4 : Math  Operator=square  OutputSignalType=auto
  Sum : Sum  Inputs=+-  SaturateOnIntegerOverflow=on
  Sum1 : Sum  Inputs=+-  SaturateOnIntegerOverflow=on
  Sum2 : Sum  Inputs=++  SaturateOnIntegerOverflow=on
  dist : Outport  Port=1  InitialOutput=0
  wires:
  Math Function2/1 -> dist/1
  y_g/1 -> Sum1/2
  x/1 -> Sum/1
  x_g/1 -> Sum/2
  y/1 -> Sum1/1
  Sum/1 -> Math Function3/1
  Math Function3/1 -> Sum2/1
  Sum1/1 -> Math Function4/1
  Math Function4/1 -> Sum2/2
  Sum2/1 -> Math Function2/1

== system HEMERO/Robots móviles/Control de robots móviles/Métodos basados en Teoría de Control/Seguimiento de caminos/Seguimiento de caminos (control lineal)/Cálculo de parámetros/Subsystem/distancia mínima1 ==
  x_camino : Inport  Port=1  PortWidth=-1  SampleTime=-1  DataType=auto
      settings: SignalType=auto
  y_camino : Inport  Port=2  PortWidth=-1  SampleTime=-1  DataType=auto
      settings: SignalType=auto
  x_vehiculo : Inport  Port=3  PortWidth=-1  SampleTime=-1  DataType=auto
      settings: SignalType=auto
  y_vehiculo : Inport  Port=4  PortWidth=-1  SampleTime=-1  DataType=auto
      settings: SignalType=auto
  Math Function2 : Math  Operator=sqrt  OutputSignalType=auto
  Math Function3 : Math  Operator=square  OutputSignalType=auto
  Math Function4 : Math  Operator=square  OutputSignalType=auto
  Minimum : dspstat/Minimum
  Sum : Sum  Inputs=+-  SaturateOnIntegerOverflow=on
  Sum1 : Sum  Inputs=+-  SaturateOnIntegerOverflow=on
  Sum2 : Sum  Inputs=++  SaturateOnIntegerOverflow=on
  d_min : Outport  Port=1  InitialOutput=0
  indice : Outport  Port=2  InitialOutput=0
  wires:
  x_camino/1 -> Sum/1
  x_vehiculo/1 -> Sum/2
  y_camino/1 -> Sum1/1
  y_vehiculo/1 -> Sum1/2
  Sum/1 -> Math Function3/1
  Math Function3/1 -> Sum2/1
  Sum1/1 -> Math Function4/1
  Math Function4/1 -> Sum2/2
  Sum2/1 -> Math Function2/1
  Math Function2/1 -> Minimum/1
  Minimum/1 -> d_min/1
  Minimum/2 -> indice/1

== system HEMERO/Robots móviles/Control de robots móviles/Métodos basados en Teoría de Control/Seguimiento de caminos/Seguimiento de caminos (control lineal)/Cálculo de parámetros/Subsystem/tres_puntos ==
  indice : Inport  Port=1  PortWidth=-1  SampleTime=-1  DataType=auto
      settings: SignalType=auto
  Constant : Constant  Value=1
  Constant1 : Constant  Value=2
  Look-Up Table : Lookup  InputValues=1:length(x_camino)  OutputValues=x_camino(1:length(x_camino))
  Look-Up Table1 : Lookup  InputValues=1:length(y_camino)  OutputValues=y_camino(1:length(y_camino))
  Look-Up Table2 : Lookup  InputValues=1:length(x_camino)  OutputValues=x_camino(1:length(x_camino))
  Look-Up Table3 : Lookup  InputValues=1:length(y_camino)  OutputValues=y_camino(1:length(y_camino))
  Look-Up Table4 : Lookup  InputValues=1:length(x_camino)  OutputValues=x_camino(1:length(x_camino))
  Look-Up Table5 : Lookup  InputValues=1:length(y_camino)  OutputValues=y_camino(1:length(y_camino))
  Sum : Sum  Inputs=++  SaturateOnIntegerOverflow=on
  Sum1 : Sum  Inputs=++  SaturateOnIntegerOverflow=on
  x_1 : Outport  Port=1
  x_2 : Outport  Port=2
  x_3 : Outport  Port=3
  y_1 : Outport  Port=4
  y_2 : Outport  Port=5
  y_3 : Outport  Port=6
  wires:
  Look-Up Table/1 -> x_1/1
  indice/1 -> Look-Up Table/1, Look-Up Table1/1, Sum/1, Sum1/1
  Constant/1 -> Sum/2
  Look-Up Table2/1 -> x_2/1
  Look-Up Table3/1 -> y_2/1
  Sum/1 -> Look-Up Table2/1, Look-Up Table3/1
  Look-Up Table1/1 -> y_1/1
  Constant1/1 -> Sum1/2
  Look-Up Table5/1 -> y_3/1
  Look-Up Table4/1 -> x_3/1
  Sum1/1 -> Look-Up Table4/1, Look-Up Table5/1

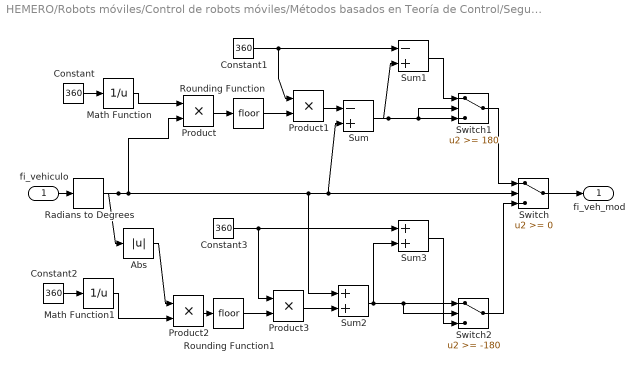
== system HEMERO/Robots móviles/Control de robots móviles/Métodos basados en Teoría de Control/Seguimiento de caminos/Seguimiento de caminos (control no lineal)/Cálculo de parámetros/Cálculo de phi gorro/Subsystem ==
  fi_vehiculo : Inport  Port=1  PortWidth=-1  SampleTime=-1  DataType=auto
      settings: SignalType=auto
  Abs : Abs
  Constant{,1..3} (4 alike) : Constant  Value=360
  Math Function : Math  Operator=reciprocal  OutputSignalType=auto
  Math Function1 : Math  Operator=reciprocal  OutputSignalType=auto
  Product{,1..3} (4 alike) : Product  Inputs=2  SaturateOnIntegerOverflow=on
  Radians to Degrees : simulink_extras/Transformations/Radians to Degrees
  Rounding Function : Rounding  Operator=floor
  Rounding Function1 : Rounding  Operator=floor
  Sum : Sum  Inputs=-+  SaturateOnIntegerOverflow=on
  Sum1 : Sum  Inputs=-+  SaturateOnIntegerOverflow=on
  Sum2 : Sum  Inputs=++  SaturateOnIntegerOverflow=on
  Sum3 : Sum  Inputs=++  SaturateOnIntegerOverflow=on
  Switch : Switch  Threshold=0
  Switch1 : Switch  Threshold=180
  Switch2 : Switch  Threshold=-180
  fi_veh_mod : Outport  Port=1
  wires:
  Radians to Degrees/1 -> Abs/1, Sum2/1, Sum/2, Switch/2, Product/2
  fi_vehiculo/1 -> Radians to Degrees/1
  Abs/1 -> Product2/1
  Sum2/1 -> Switch2/2, Switch2/1, Sum3/2
  Sum3/1 -> Switch2/3
  Product2/1 -> Rounding Function1/1
  Math Function1/1 -> Product2/2
  Constant2/1 -> Math Function1/1
  Product3/1 -> Sum2/2
  Rounding Function1/1 -> Product3/2
  Switch2/1 -> Switch/3
  Constant3/1 -> Sum3/1, Product3/1
  Sum1/1 -> Switch1/1
  Sum/1 -> Switch1/2, Switch1/3, Sum1/2
  Constant1/1 -> Sum1/1, Product1/1
  Product1/1 -> Sum/1
  Rounding Function/1 -> Product1/2
  Product/1 -> Rounding Function/1
  Constant/1 -> Math Function/1
  Math Function/1 -> Product/1
  Switch1/1 -> Switch/1
  Switch/1 -> fi_veh_mod/1

== system HEMERO/Robots móviles/Control de robots móviles/Métodos basados en Teoría de Control/Seguimiento de caminos/Seguimiento de caminos (control no lineal)/Cálculo de parámetros/Cálculo de phi gorro/Subsystem1 ==
  indice : Inport  Port=1  PortWidth=-1  SampleTime=-1  DataType=auto
      settings: SignalType=auto
  Constant : Constant  Value=90
  Constant1 : Constant  Value=360
  Look-Up Table : Lookup  InputValues=1:length(der_x)  OutputValues=der_x(1:length(der_x))
  Look-Up Table1 : Lookup  InputValues=1:length(der_y)  OutputValues=der_y(1:length(der_y))
  Radians to Degrees : simulink_extras/Transformations/Radians to Degrees
  Sum : Sum  Inputs=+-  SaturateOnIntegerOverflow=on
  Sum1 : Sum  Inputs=++  SaturateOnIntegerOverflow=on
  Switch : Switch  Threshold=-180
  Trigonometric Function : Trigonometry  Operator=atan2  OutputSignalType=auto
  fi_camino : Outport  Port=1
  wires:
  indice/1 -> Look-Up Table/1, Look-Up Table1/1
  Switch/1 -> fi_camino/1
  Sum1/1 -> Switch/3
  Sum/1 -> Switch/2, Sum1/1, Switch/1
  Constant1/1 -> Sum1/2
  Constant/1 -> Sum/2
  Radians to Degrees/1 -> Sum/1
  Trigonometric Function/1 -> Radians to Degrees/1
  Look-Up Table/1 -> Trigonometric Function/2
  Look-Up Table1/1 -> Trigonometric Function/1
